simulink model "FOC_ClosedLoop"  (R2023a)
settings: Solver=FixedStepAuto  StartTime=0.0  StopTime=0.5  FixedStep=0.0001  RelTol=1e-3
settings Model: Creator=HP  LastModifiedBy=HP

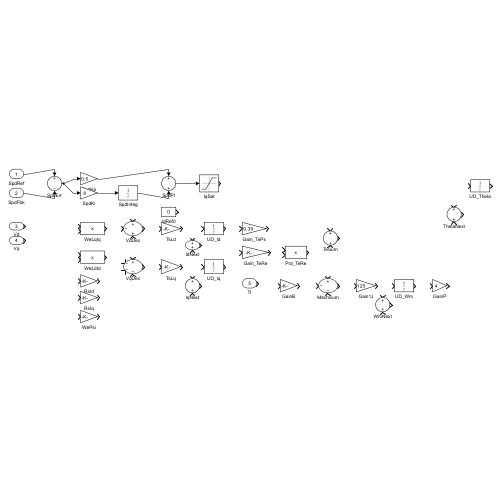
[thumbnail: Simulink's stored preview of the top-level diagram]
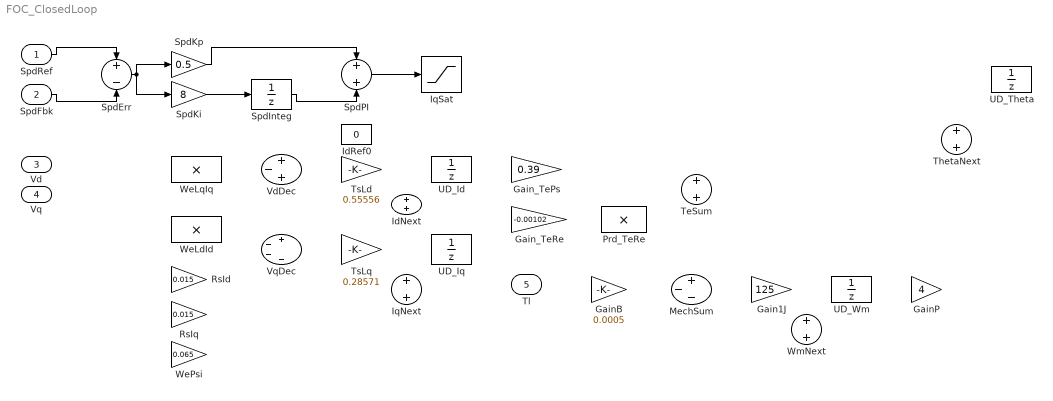
== system FOC_ClosedLoop ==
  SpdRef : Inport
  SpdFbk : Inport  Port=2
  Vd : Inport  Port=3
  Vq : Inport  Port=4
  Tl : Inport  Port=5
  Gain1J : Gain  Gain=125
  GainB : Gain  Gain=0.0005
  GainP : Gain  Gain=4
  Gain_TePs : Gain  Gain=0.39
  Gain_TeRe : Gain  Gain=-0.00102
  IdNext : Sum
  IdRef0 : Constant  Value=0
  IqNext : Sum
  IqSat : Saturate  UpperLimit=400  LowerLimit=-400
  MechSum : Sum  Inputs=+--
  Prd_TeRe : Product  Inputs=**
  RsId : Gain  Gain=0.015
  RsIq : Gain  Gain=0.015
  SpdErr : Sum  Inputs=+-
  SpdInteg : UnitDelay  SampleTime=0.0001  HasFrameUpgradeWarning=on
  SpdKi : Gain  Gain=8
  SpdKp : Gain  Gain=0.5
  SpdPI : Sum
  TeSum : Sum
  ThetaNext : Sum
  TsLd : Gain  Gain=0.55556
  TsLq : Gain  Gain=0.28571
  UD_Id : UnitDelay  SampleTime=0.0001  HasFrameUpgradeWarning=on
  UD_Iq : UnitDelay  SampleTime=0.0001  HasFrameUpgradeWarning=on
  UD_Theta : UnitDelay  SampleTime=0.0001  HasFrameUpgradeWarning=on
  UD_Wm : UnitDelay  SampleTime=0.0001  HasFrameUpgradeWarning=on
  VdDec : Sum  Inputs=+-+
  VqDec : Sum  Inputs=+---
  WeLdId : Product  Inputs=**
  WeLqIq : Product  Inputs=**
  WePsi : Gain  Gain=0.065
  WmNext : Sum
  wires:
  SpdRef/1 -> SpdErr/1
  SpdFbk/1 -> SpdErr/2
  SpdErr/1 -> SpdKp/1, SpdKi/1
  SpdKi/1 -> SpdInteg/1
  SpdInteg/1 -> SpdPI/2
  SpdKp/1 -> SpdPI/1
  SpdPI/1 -> IqSat/1
